simulink model "AdaptiveCompTorque"  (R2019b)
settings: Solver=VariableStepAuto  StartTime=0.0  StopTime=10.0  RelTol=1e-3
undefined symbols (not defined in the file): a0, a1, a2, a3, parameter, x_endEff_D
libraries: simulink x1
settings Model: Creator=ariannagasparri  LastModifiedBy=ariannagasparri

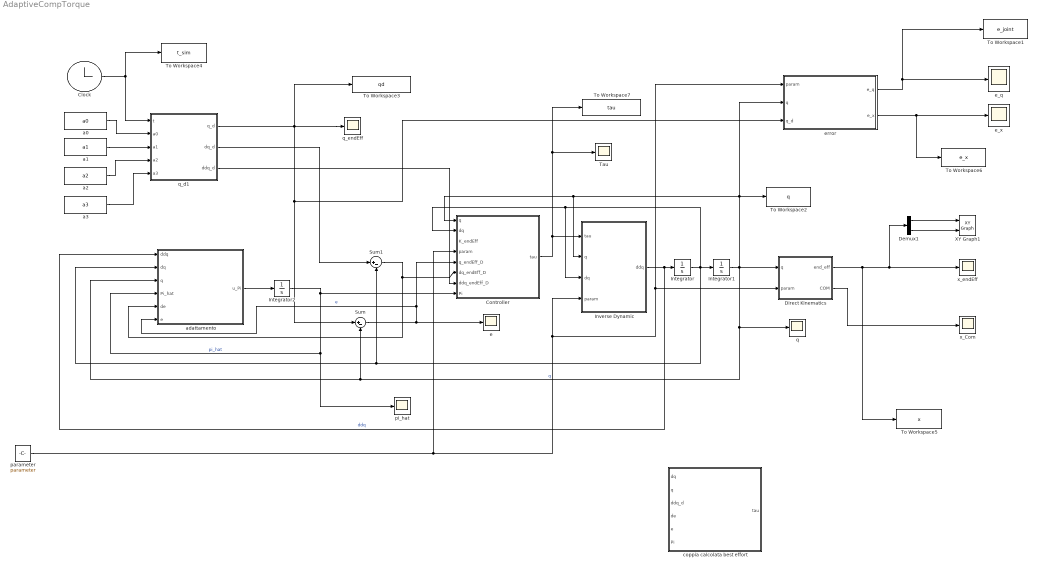
== system AdaptiveCompTorque ==
  Clock : Clock
  Controller : MATLAB Function  TreatAsAtomicUnit=on
  Demux1 : Demux  Outputs=3
  "Direct Kinematics " : MATLAB Function  TreatAsAtomicUnit=on
  Integrator : Integrator
  Integrator1 : Integrator  InitialCondition=-pi/2
  Integrator2 : Integrator  InitialCondition=[0.5; 4.9]
  "Inverse Dynamic " : MATLAB Function  TreatAsAtomicUnit=on
  Sum : Sum  Inputs=|+-
  Sum1 : Sum  Inputs=|+-
  Tau : Scope
  To Workspace1 : ToWorkspace  VariableName=e_joint  SaveFormat=Structure With Time  SampleTime=-1
  To Workspace2 : ToWorkspace  VariableName=q  SaveFormat=Structure With Time  SampleTime=-1
  To Workspace3 : ToWorkspace  VariableName=qd  SaveFormat=Structure With Time  SampleTime=-1
  To Workspace4 : ToWorkspace  VariableName=t_sim  SaveFormat=Structure With Time  SampleTime=-1
  To Workspace5 : ToWorkspace  VariableName=x  SaveFormat=Structure With Time  SampleTime=-1
  To Workspace6 : ToWorkspace  VariableName=e_x  SaveFormat=Structure With Time  SampleTime=-1
  To Workspace7 : ToWorkspace  VariableName=tau  SaveFormat=Structure With Time  SampleTime=-1
  XY Graph1 : simulink/Sinks/XY Graph  xmin=x_endEff_D(1)-2  xmax=x_endEff_D(1)+2  ymin=x_endEff_D(3)-2  ymax=x_endEff_D(3)+2  st=-1
  a0 : Constant  Value=a0
  a1 : Constant  Value=a1
  a2 : Constant  Value=a2
  a3 : Constant  Value=a3
  adattamento : MATLAB Function  TreatAsAtomicUnit=on
  coppia calcolata best effort : MATLAB Function  TreatAsAtomicUnit=on
  e : Scope
  e_q : Scope
  e_x : Scope
  error : MATLAB Function  TreatAsAtomicUnit=on
  "parameter " : Constant  Value=parameter
  pi_hat : Scope
  q : Scope
  q_d1 : MATLAB Function  TreatAsAtomicUnit=on
  q_endEff : Scope
  x_Com : Scope
  x_endEff : Scope
  wires:
  Integrator/1 -> Controller/2(dq), "Inverse Dynamic "/3(dq), Integrator1/1, adattamento/2(dq), Sum1/2
  adattamento/1(u_Pi) -> Integrator2/1
  Sum/1 -> Controller/5(q_endEff_D), adattamento/6(e), e/1  "e"
  Sum1/1 -> Controller/6(dq_endEff_D), adattamento/5(de)
  Integrator2/1 -> Controller/8(Pi), pi_hat/1, adattamento/4(Pi_hat)  "pi_hat"
  Integrator1/1 -> "Direct Kinematics "/1(q), Sum/2, adattamento/3(q), q/1, error/2(q), Controller/1(q), "Inverse Dynamic "/2(q), To Workspace2/1  "q"
  "Inverse Dynamic "/1(ddq) -> Integrator/1, adattamento/1(ddq)  "ddq"
  a3/1 -> q_d1/5(a3)
  q_d1/2(dq_d) -> Sum1/1
  a0/1 -> q_d1/2(a0)
  q_d1/3(ddq_d) -> Controller/7(ddq_endEff_D)
  Clock/1 -> q_d1/1(t), To Workspace4/1
  a1/1 -> q_d1/3(a1)
  a2/1 -> q_d1/4(a2)
  "Direct Kinematics "/2(COM) -> x_Com/1
  Demux1/1 -> XY Graph1/1
  Demux1/3 -> XY Graph1/2
  "Direct Kinematics "/1(end_eff) -> To Workspace5/1, Demux1/1, x_endEff/1
  "parameter "/1 -> Controller/4(param), "Direct Kinematics "/2(param), error/1(param), "Inverse Dynamic "/4(param)
  q_d1/1(q_d) -> error/3(q_d), Sum/1, q_endEff/1, To Workspace3/1
  error/2(e_x) -> To Workspace6/1, e_x/1
  error/1(e_q) -> To Workspace1/1, e_q/1
  Controller/1(tau) -> "Inverse Dynamic "/1(tau), Tau/1, To Workspace7/1

== matlab function AdaptiveCompTorque/coppia calcolata best effort ==
  data: dq input; q input; ddq_d input; tau output; de input; e input; Pi input
function tau = dyn( dq, q, ddq_d, de, e, Pi)

% m = 1;      % kg massa del pendolo
% l = 1;      % m lunghezza del pendolo
% g  = 9.81;  % kg*m/s^2 acc di gravita'

% Pi =  [l^2*m ;  g*l*m ]

% Pi =  [1 ;  9,81 ]

Kp = 10;
Kv = 10;

% tau = (m*l^2)*(ddq_d + Kv*de + Kp*e) + g*m*l*cos(q);

tau = Pi(1)*(ddq_d + Kv*de + Kp*e) + Pi(2)*cos(q);

== matlab function AdaptiveCompTorque/Controller ==
  data: q input; dq input; K_endEff input; tau output; param input; q_endEff_D input; dq_endEff_D input; ddq_endEff_D input; Pi input
function tau  = x_now(q, dq, K_endEff, param, q_endEff_D, dq_endEff_D, ddq_endEff_D, Pi)

%     G = G_f(q_endEff_D,param);
%     B = B_f(q_endEff_D, param);
%     C = C_f(q_endEff_D, dq_endEff_D, param);

    G = G_f(q, param);
    B = B_f(q, param);
    C = C_f(q, dq, param);
    
    Kp_endEff = K_endEff(1);
    Kd_endEff = K_endEff(2);
    %Kp_endEff = K_endEff(1:6,1:6);
    %Kd_endEff = K_endEff(1:6,7:12);
    
    %% controllo priorità di task
    %J_endEff_pinv = pinv(J_endEff);
    %J_COM = JacobianCom(param,q);
    %P_endEff = (eye(6) - J_endEff_pinv*J_endEff); %PROIEZIONE NULLO
       
    %e_COM = x_COM_D - x_COM;
    
    %tau = - Kd_endEff*dq + J_endEff_pinv*Kp_endEff*e_endEff;% + pinv(J_COM*P_endEff)*Kp_COM*e_COM;
    
    %% controllo Diretto
    
    e_endEff = q_endEff_D - q;
    de_endEff = dq_endEff_D - dq;
    
%     tau = Kp_endEff*e_endEff + Kd_endEff*de_endEff + G + C*dq + B*ddq_endEff_D;
    tau = Pi(1)*(ddq_endEff_D + Kd_endEff*de_endEff + Kp_endEff*e_endEff) + Pi(2)*cos(q);
    
end

== matlab function AdaptiveCompTorque/adattamento ==
  data: ddq input; dq input; q input; u_Pi output; Pi_hat input; de input; e input
function u_Pi = adattamento(ddq, dq, q, Pi_hat, de, e)

% Pi =  [l^2*m ;  g*l*m ]

R = diag([10 10]);
Y = [ddq, cos(q)];
M_hat = Pi_hat(1);
B = [0;1];
P = diag([3 2]);
x = [de; e];

u_Pi = inv(R) * Y' * inv(M_hat) * B' * P * x;

== matlab function AdaptiveCompTorque/Inverse Dynamic  ==
  data: tau input; q input; dq input; ddq output; param input
function ddq = inverseDynamic(tau,q,dq,param)

    B = B_f(q, param);
    G = G_f(q, param);
    C = C_f(q, dq, param);
    
    ddq = B\(tau - G - C*dq);

end

== matlab function AdaptiveCompTorque/Direct Kinematics  ==
  data: q input; end_eff output; param input; COM output
function [end_eff, COM] = DirectK(q,param)


    [Pcom, Etip,T00,T01,T12,T23,T34,T45,T56] =  forwardKinematics(param, q);
    
    
    end_eff = Etip(1:3,4);
    COM = Pcom;
    
end

== matlab function AdaptiveCompTorque/q_d1 ==
  data: t input; q_d output; dq_d output; ddq_d output; a0 input; a1 input; a2 input; a3 input
function [q_d,dq_d,ddq_d] = desiderable_q(t, a0,a1,a2,a3)

    [q_d, dq_d, ddq_d] = vettoreq(a0,a1,a2,a3,t);
    
end

== matlab function AdaptiveCompTorque/error ==
  data: param input; q input; e_q output; q_d input; e_x output
function [e_q, e_x]  = error(param, q, q_d)
    

%     [~, Etip,~,~,~,~,~,~,~] =  forwardKinematics(param, q*pi/180);
%     [~, Etip_d,~,~,~,~,~,~,~] =  forwardKinematics(param, q_d*pi/180);  

    [~, Etip,~,~,~,~,~,~,~] =  forwardKinematics(param, q);
    [~, Etip_d,~,~,~,~,~,~,~] =  forwardKinematics(param, q_d);  

    e_x = Etip_d(1:3,4) - Etip(1:3,4);

    e_q = q_d - q;
    
end
